simulink model "model2_Zk"  (R2019a)
settings: Solver=VariableStepAuto  StartTime=0.0  StopTime=10  RelTol=1e-3
values from neighbouring files (symbols this model uses):
  AngleW = ExoD.A(3,1:3)/Ks    [LoadDatas.m]    (also in exportCpp.mat = [-1.9997000284e-07 4.24506510462e-08 0.01]; simulation_2.m)
  Exo2 = d2c(Exo2,'tustin')    [LoadDatas.m]    (also in model2_m.m = d2c(Exo2d,'tustin'))
  Wcmd = tf(1)    [LoadDatas.m]    (also in model2_m.m = Wcmd*1.7)
  We1 = tf([0.03448 20.69], [1 0.72])    [LoadDatas.m]    (also in model2_m.m)
  Wnoise = tf(1)    [LoadDatas.m]    (also in model2_m.m = Wnoise)
libraries: simulink x2
settings Model: Creator=YecidMoreno  LastModifiedBy=YecidMoreno
settings SolverCC: AlgebraicLoopSolver=LineSearch

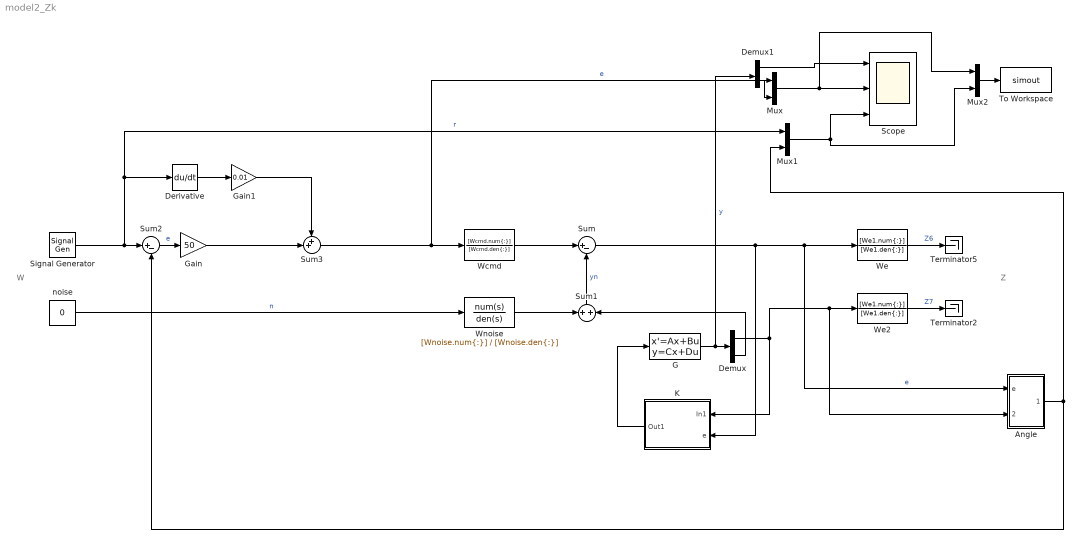
== system model2_Zk ==
  note: Z
  note: W
  Angle : Subsystem
  Demux : Demux  Outputs=2
  Demux1 : Demux  Outputs=2
  Derivative : Derivative
  G : StateSpace  A=Exo2.A  B=Exo2.B  C=Exo2.C  D=Exo2.D  InitialCondition=[]
  Gain : Gain  Gain=50
  Gain1 : Gain  Gain=0.01
  K : Subsystem
  Mux : Mux  Inputs=2
  Mux1 : Mux  Inputs=2
  Mux2 : Mux  Inputs=2
  Scope : Scope  NumInputPorts=3
  Signal Generator : SignalGenerator  Amplitude=0.1
  Sum : Sum  Inputs=|+-  SaturateOnIntegerOverflow=on
  Sum1 : Sum  SaturateOnIntegerOverflow=on
  Sum2 : Sum  Inputs=|+-  SaturateOnIntegerOverflow=on
  Sum3 : Sum  Inputs=++|  SaturateOnIntegerOverflow=on
  Terminator2 : Terminator
  Terminator5 : Terminator
  To Workspace : ToWorkspace  VariableName=simout  SaveFormat=Timeseries  SampleTime=-1
  Wcmd : TransferFcn  Numerator=[Wcmd.num{:}]  Denominator=[Wcmd.den{:}]
  We : TransferFcn  Numerator=[We1.num{:}]  Denominator=[We1.den{:}]
  We2 : TransferFcn  Numerator=[We1.num{:}]  Denominator=[We1.den{:}]
  Wnoise : TransferFcn  Numerator=[Wnoise.num{:}]  Denominator=[Wnoise.den{:}]
  noise : Constant  Value=0
  wires:
  noise/1 -> Wnoise/1  "n"
  We/1 -> Terminator5/1  "Z6"
  Sum1/1 -> Sum/2  "yn"
  Demux/1 -> K/1(In1), Angle/2(In2), We2/1
  G/1 -> Demux1/1, Demux/1  "y"
  Wcmd/1 -> Sum/1
  Sum/1 -> K/2(e), Angle/1(e), We/1  "e"
  We2/1 -> Terminator2/1  "Z7"
  K/1(Out1) -> G/1
  Wnoise/1 -> Sum1/1
  Demux/2 -> Sum1/2
  Demux1/1 -> Scope/1
  Demux1/2 -> Mux/2
  Mux/1 -> Mux2/1, Scope/2
  Angle/1(Out1) -> Mux1/2, Sum2/2
  Signal Generator/1 -> Mux1/1, Derivative/1, Sum2/1  "r"
  Sum2/1 -> Gain/1  "e"
  Mux1/1 -> Scope/3, Mux2/2
  Sum3/1 -> Mux/1, Wcmd/1  "e"
  Gain/1 -> Sum3/2
  Derivative/1 -> Gain1/1
  Gain1/1 -> Sum3/1
  Mux2/1 -> To Workspace/1

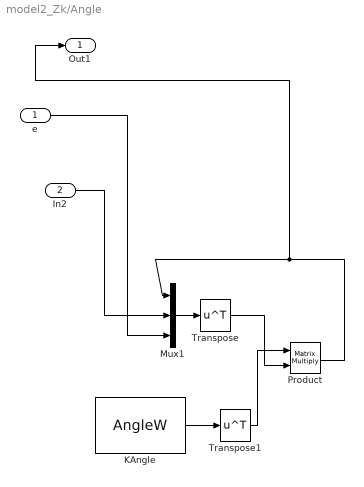
== system model2_Zk/Angle ==
  e : Inport
  In2 : Inport  Port=2
  KAngle : Constant  Value=AngleW
  Mux1 : Mux  Inputs=3
  Product : Product  Multiplication=Matrix(*)
  Transpose : Math  Operator=transpose  SaturateOnIntegerOverflow=on
  Transpose1 : Math  Operator=transpose  SaturateOnIntegerOverflow=on
  Out1 : Outport
  wires:
  Product/1 -> Out1/1, Mux1/1
  Mux1/1 -> Transpose/1
  KAngle/1 -> Transpose1/1
  e/1 -> Mux1/3
  In2/1 -> Mux1/2
  Transpose1/1 -> Product/1
  Transpose/1 -> Product/2

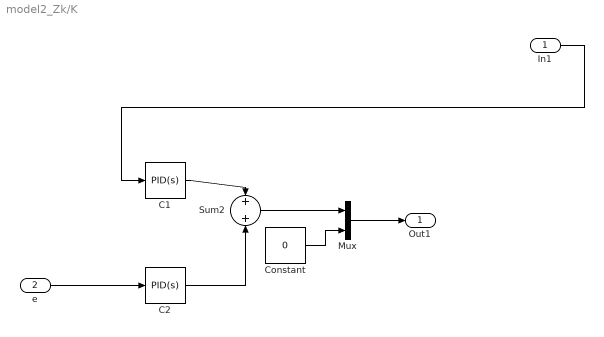
== system model2_Zk/K ==
  In1 : Inport
  e : Inport  Port=2
  C1 : simulink/Continuous/PID Controller  Controller=PID  Form=Parallel  TimeDomain=Continuous-time  SampleTime=-1  IntegratorMethod=Forward Euler  FilterMethod=Forward Euler  ControllerParametersSource=internal  P=-176.7083  I=-162.8012  D=18.3293  UseFilter=on  N=10  TunerSelectOption=Transfer Function Based (PID Tuner App)  InitialConditionSource=internal  InitialConditionForIntegrator=0  InitialConditionForFilter=0  DifferentiatorICPrevScaledInput=0  ExternalReset=none  TrackingMode=off  Kt=1  LimitOutput=off  UpperSaturationLimit=inf  LowerSaturationLimit=-inf  LinearizeAsGain=off  AntiWindupMode=none  Kb=1  POutMin=[]  POutMax=[]  IOutMin=[]  IOutMax=[]  DOutMin=[]  DOutMax=[]  NOutMin=[]  NOutMax=[]  SumOutMin=[]  SumOutMax=[]  SaturationOutMin=[]  SaturationOutMax=[]  PParamMin=[]  PParamMax=[]  IParamMin=[]  IParamMax=[]  DParamMin=[]  DParamMax=[]  NParamMin=[]  NParamMax=[]  KbParamMin=[]  KbParamMax=[]  KtParamMin=[]  KtParamMax=[]  KbOutMin=[]  KbOutMax=[]  KtOutMin=[]  KtOutMax=[]  IntegratorOutMin=[]  IntegratorOutMax=[]  FilterOutMin=[]  FilterOutMax=[]  SumI1OutMin=[]  SumI1OutMax=[]  SumI2OutMin=[]  SumI2OutMax=[]  SumI3OutMin=[]  SumI3OutMax=[]  SumI4OutMin=[]  SumI4OutMax=[]  SumDOutMin=[]  SumDOutMax=[]  DifferentiatorOutMin=[]  DifferentiatorOutMax=[]  FilterDiffOutCoefMin=[]  FilterDiffOutCoefMax=[]  ReciprocalOutMin=[]  ReciprocalOutMax=[]  SumDenOutMin=[]  SumDenOutMax=[]  SumNumOutMin=[]  SumNumOutMax=[]  DivideOutMin=[]  DivideOutMax=[]  IntegratorContinuousStateAttributes=''  IntegratorStateMustResolveToSignalObject=off  IntegratorRTWStateStorageClass=Auto  FilterContinuousStateAttributes=''  FilterStateMustResolveToSignalObject=off  FilterRTWStateStorageClass=Auto  ParallelPVariant=InternalParameters  IdealPVariant=Disabled  IVariant=InternalParameters  DVariant=InternalParameters  IntegratorVariant=Continuous  SatVariant=Disabled  AWVariant=Passthrough  PCopyVariant=Disabled  TRVariant=Disabled  FdbkBlocksVariant=Forward  IdealPFdbkVariant=Disabled  SatFdbkVariant=Disabled  DerivativeFilterVariant=ContFilter  NVariant=InternalParameters  NCopyVariant=Disabled  FilterICVariant=InternalICsFilter  IntegratorICVariant=InternalICs  ExternalResetVariant=Disabled  TRSumVariant=Passthrough  SumFdbkVariant=Disabled  SumVariant=Sum_PID
  C2 : simulink/Continuous/PID Controller  Controller=PID  Form=Parallel  TimeDomain=Continuous-time  SampleTime=-1  IntegratorMethod=Forward Euler  FilterMethod=Forward Euler  ControllerParametersSource=internal  P=1403.7416  I=0.00024242  D=113.8358  UseFilter=on  N=100  TunerSelectOption=Frequency Response Based  InitialConditionSource=internal  InitialConditionForIntegrator=0  InitialConditionForFilter=0  DifferentiatorICPrevScaledInput=0  ExternalReset=none  TrackingMode=off  Kt=1  LimitOutput=off  UpperSaturationLimit=inf  LowerSaturationLimit=-inf  LinearizeAsGain=off  AntiWindupMode=none  Kb=1  POutMin=[]  POutMax=[]  IOutMin=[]  IOutMax=[]  DOutMin=[]  DOutMax=[]  NOutMin=[]  NOutMax=[]  SumOutMin=[]  SumOutMax=[]  SaturationOutMin=[]  SaturationOutMax=[]  PParamMin=[]  PParamMax=[]  IParamMin=[]  IParamMax=[]  DParamMin=[]  DParamMax=[]  NParamMin=[]  NParamMax=[]  KbParamMin=[]  KbParamMax=[]  KtParamMin=[]  KtParamMax=[]  KbOutMin=[]  KbOutMax=[]  KtOutMin=[]  KtOutMax=[]  IntegratorOutMin=[]  IntegratorOutMax=[]  FilterOutMin=[]  FilterOutMax=[]  SumI1OutMin=[]  SumI1OutMax=[]  SumI2OutMin=[]  SumI2OutMax=[]  SumI3OutMin=[]  SumI3OutMax=[]  SumI4OutMin=[]  SumI4OutMax=[]  SumDOutMin=[]  SumDOutMax=[]  DifferentiatorOutMin=[]  DifferentiatorOutMax=[]  FilterDiffOutCoefMin=[]  FilterDiffOutCoefMax=[]  ReciprocalOutMin=[]  ReciprocalOutMax=[]  SumDenOutMin=[]  SumDenOutMax=[]  SumNumOutMin=[]  SumNumOutMax=[]  DivideOutMin=[]  DivideOutMax=[]  IntegratorContinuousStateAttributes=''  IntegratorStateMustResolveToSignalObject=off  IntegratorRTWStateStorageClass=Auto  FilterContinuousStateAttributes=''  FilterStateMustResolveToSignalObject=off  FilterRTWStateStorageClass=Auto  ParallelPVariant=InternalParameters  IdealPVariant=Disabled  IVariant=InternalParameters  DVariant=InternalParameters  IntegratorVariant=Continuous  SatVariant=Disabled  AWVariant=Passthrough  PCopyVariant=Disabled  TRVariant=Disabled  FdbkBlocksVariant=Forward  IdealPFdbkVariant=Disabled  SatFdbkVariant=Disabled  DerivativeFilterVariant=ContFilter  NVariant=InternalParameters  NCopyVariant=Disabled  FilterICVariant=InternalICsFilter  IntegratorICVariant=InternalICs  ExternalResetVariant=Disabled  TRSumVariant=Passthrough  SumFdbkVariant=Disabled  SumVariant=Sum_PID
  Constant : Constant  Value=0
  Mux : Mux  Inputs=2
  Sum2 : Sum  SaturateOnIntegerOverflow=on
  Out1 : Outport
  wires:
  C2/1 -> Sum2/2
  Constant/1 -> Mux/2
  C1/1 -> Sum2/1
  e/1 -> C2/1
  In1/1 -> C1/1
  Sum2/1 -> Mux/1
  Mux/1 -> Out1/1
